simulink model "SigProcess"  (R2022b)
settings: Solver=FixedStepDiscrete  StartTime=0.0  StopTime=10.0  FixedStep=0.001  RelTol=1e-3
undefined symbols (not defined in the file): cClCddAdc_D_u16ADNum, cClCddAdc_D_u8FilterType, cClCddAdc_D_u8RawValueNum, cTmAfCtrl_Te_s32ShttrPosnColdOnHp
libraries: simulink x132
(part 1 of 7)
settings Model: PacingRate=0.500000  Creator=blue.ge  LastModifiedBy=blue.ge
settings OptimizationCC: DefaultParameterBehavior=Inlined  DefaultUnderspecifiedDataType=single  InlineInvariantSignals=on  EnhancedBackFolding=on  StrengthReduction=on  StateBitsets=on  DataBitsets=on  ZeroExternalMemoryAtStartup=off  ZeroInternalMemoryAtStartup=off  EfficientFloat2IntCast=on  LifeSpan=inf  EfficientTunableParamExpr=on
settings DebuggingCC: ConsistencyChecking=error  SignalInfNanChecking=warning  SignalRangeChecking=warning  AlgebraicLoopMsg=error  ArtificialAlgebraicLoopMsg=error  SaveWithDisabledLinksMsg=none  SaveWithParameterizedLinksMsg=none  SignalResolutionControl=TryResolveAll  BlockPriorityViolationMsg=error  SolverPrmCheckMsg=error  SingleTaskRateTransMsg=error  SigSpecEnsureSampleTimeMsg=error  CheckMatrixSingularityMsg=error  ParameterOverflowMsg=warning  ParameterUnderflowMsg=error  ParameterTunabilityLossMsg=error  UnderSpecifiedDataTypeMsg=warning  UnnecessaryDatatypeConvMsg=warning  VectorMatrixConversionMsg=error  SignalLabelMismatchMsg=warning  UnconnectedLineMsg=error  UniqueDataStoreMsg=error  BusObjectLabelMismatch=error  RootOutportRequireBusObject=error  AllowSymbolicDim=off  ModelReferenceIOMsg=error  ModelReferenceIOMismatchMessage=error  UnknownTsInhSupMsg=error  ModelReferenceDataLoggingMessage=error  ModelReferenceNoExplicitFinalValueMsg=error  StateNameClashWarn=warning  StrictBusMsg=ErrorOnBusTreatedAsVector  NonBusSignalsTreatedAsBus=warning  SFTemporalDelaySmallerThanSampleTimeDiag=error  SFMachineParentedDataDiag=warning  VariantConditionMismatch=warning
settings HardwareCC: ProdBitPerPointer=32  ProdBitPerSizeT=32  ProdBitPerPtrDiffT=32  ProdLargestAtomicInteger=Long  ProdWordSize=32  ProdLongLongMode=on  ProdHWDeviceType=Infineon->TriCore
settings ModelReferenceCC: EnableRefExpFcnMdlSchedulingChecks=on  EnableParallelModelReferenceBuilds=on  ParallelModelReferenceMATLABWorkerInit=Copy Base Workspace  ModelReferenceNumInstancesAllowed=Single  PropagateSignalLabelsOutOfModel=off
settings SFSimCC: MATLABDynamicMemAlloc=off  CustomCodeUndefinedFunction=UseInterfaceOnly
settings RTWCC: Description=AUTOSAR  SystemTargetFile=autosar.tlc  GenCodeOnly=on  TemplateMakefile=ert_default_tmf
settings CodeAppCC: GenerateComments=off  IgnoreCustomStorageClasses=off  MaxIdLength=100  OperatorAnnotations=on  SimulinkDataObjDesc=on  SFDataObjDesc=on  MangleLength=10  CustomSymbolStrGlobalVar=global_$R$N$M  CustomSymbolStrType=$N$R$M  CustomSymbolStrBlkIO=local_$N$M  CustomSymbolStrTmpVar=temp_$N$M  SimulinkBlockComments=off
settings STFCustomTargetCC: TargetLangStandard=C99 (ISO)  MultiwordLength=256  ParMdlRefBuildCompliant=on  CompOptLevelCompliant=on  IncludeMdlTerminateFcn=off  CombineOutputUpdateFcns=on  SuppressErrorStatus=on  ERTCustomFileBanners=on  SupportNonFinite=off  SupportComplex=off  SupportContinuousTime=off  SupportNonInlinedSFcns=off  RemoveResetFunc=on  MATLABClassNameForMDSCustomization=Simulink.SoftwareTarget.ERTCustomization  AutosarCompliant=on  UseToolchainInfoCompliant=on  LookupTableObjectStructAxisOrder=2,1,3,4,...  LUTObjectStructOrderEvenSpacing=Size,Table,Breakpoints  SystemTargetFile=autosar.tlc
settings ERTTargetCC: TargetLangStandard=C99 (ISO)  ConcurrentExecutionCompliant=off  IncludeMdlTerminateFcn=off  SuppressErrorStatus=on  SupportNonFinite=off  SupportComplex=off  ModelStepFunctionPrototypeControlCompliant=off  CPPClassGenCompliant=off  AutosarCompliant=on  LookupTableObjectStructAxisOrder=2,1,3,4,...  LUTObjectStructOrderEvenSpacing=Size,Table,Breakpoints  GenerateASAP2=on  InlinedParameterPlacement=NonHierarchical  ERTCustomFileTemplate=example_file_process.tlc  ERTFilePackagingFormat=Compact  ConvertIfToSwitch=off

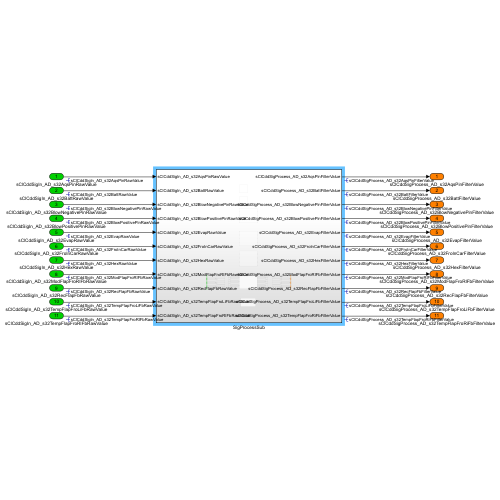
[thumbnail: Simulink's stored preview of the top-level diagram]
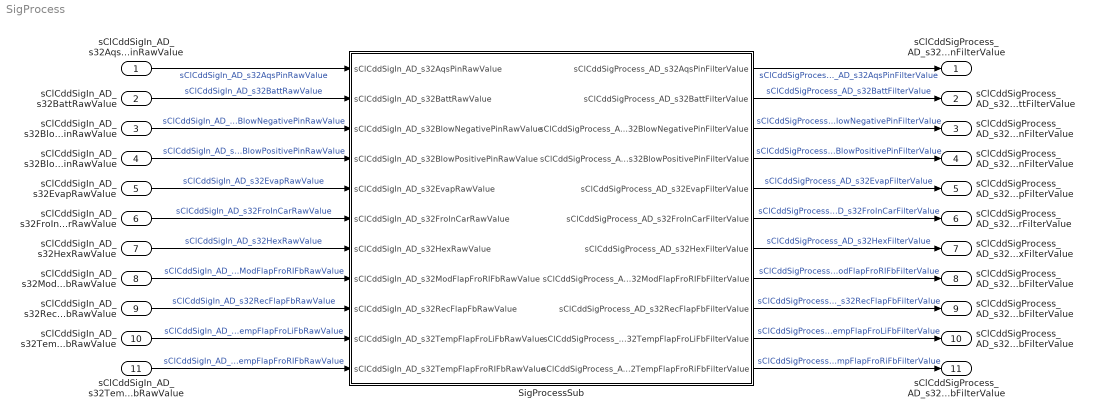
== system SigProcess ==
  sClCddSigIn_AD_s32AqsPinRawValue : Inport  OutDataTypeStr=single
  sClCddSigIn_AD_s32BattRawValue : Inport  Port=2  OutDataTypeStr=single
  sClCddSigIn_AD_s32BlowNegativePinRawValue : Inport  Port=3  OutDataTypeStr=single
  sClCddSigIn_AD_s32BlowPositivePinRawValue : Inport  Port=4  OutDataTypeStr=single
  sClCddSigIn_AD_s32EvapRawValue : Inport  Port=5  OutDataTypeStr=single
  sClCddSigIn_AD_s32FroInCarRawValue : Inport  Port=6  OutDataTypeStr=single
  sClCddSigIn_AD_s32HexRawValue : Inport  Port=7  OutDataTypeStr=single
  sClCddSigIn_AD_s32ModFlapFroRIFbRawValue : Inport  Port=8  OutDataTypeStr=single
  sClCddSigIn_AD_s32RecFlapFbRawValue : Inport  Port=9  OutDataTypeStr=single
  sClCddSigIn_AD_s32TempFlapFroLiFbRawValue : Inport  Port=10  OutDataTypeStr=single
  sClCddSigIn_AD_s32TempFlapFroRIFbRawValue : Inport  Port=11  OutDataTypeStr=single
  SigProcessSub : Subsystem
  sClCddSigProcess_AD_s32AqsPinFilterValue : Outport  OutDataTypeStr=single
  sClCddSigProcess_AD_s32BattFilterValue : Outport  Port=2  OutDataTypeStr=single
  sClCddSigProcess_AD_s32BlowNegativePinFilterValue : Outport  Port=3  OutDataTypeStr=single
  sClCddSigProcess_AD_s32BlowPositivePinFilterValue : Outport  Port=4  OutDataTypeStr=single
  sClCddSigProcess_AD_s32EvapFilterValue : Outport  Port=5  OutDataTypeStr=single
  sClCddSigProcess_AD_s32FroInCarFilterValue : Outport  Port=6  OutDataTypeStr=single
  sClCddSigProcess_AD_s32HexFilterValue : Outport  Port=7  OutDataTypeStr=single
  sClCddSigProcess_AD_s32ModFlapFroRIFbFilterValue : Outport  Port=8  OutDataTypeStr=single
  sClCddSigProcess_AD_s32RecFlapFbFilterValue : Outport  Port=9  OutDataTypeStr=single
  sClCddSigProcess_AD_s32TempFlapFroLiFbFilterValue : Outport  Port=10  OutDataTypeStr=single
  sClCddSigProcess_AD_s32TempFlapFroRiFbFilterValue : Outport  Port=11  OutDataTypeStr=single
  wires:
  sClCddSigIn_AD_s32AqsPinRawValue/1 -> SigProcessSub/1(sClCddSigIn_AD_s32AqsPinRawValue)  "sClCddSigIn_AD_s32AqsPinRawValue"
  sClCddSigIn_AD_s32BattRawValue/1 -> SigProcessSub/2(sClCddSigIn_AD_s32BattRawValue)  "sClCddSigIn_AD_s32BattRawValue"
  sClCddSigIn_AD_s32BlowNegativePinRawValue/1 -> SigProcessSub/3(sClCddSigIn_AD_s32BlowNegativePinRawValue)  "sClCddSigIn_AD_s32BlowNegativePinRawValue"
  sClCddSigIn_AD_s32BlowPositivePinRawValue/1 -> SigProcessSub/4(sClCddSigIn_AD_s32BlowPositivePinRawValue)  "sClCddSigIn_AD_s32BlowPositivePinRawValue"
  sClCddSigIn_AD_s32EvapRawValue/1 -> SigProcessSub/5(sClCddSigIn_AD_s32EvapRawValue)  "sClCddSigIn_AD_s32EvapRawValue"
  sClCddSigIn_AD_s32FroInCarRawValue/1 -> SigProcessSub/6(sClCddSigIn_AD_s32FroInCarRawValue)  "sClCddSigIn_AD_s32FroInCarRawValue"
  sClCddSigIn_AD_s32HexRawValue/1 -> SigProcessSub/7(sClCddSigIn_AD_s32HexRawValue)  "sClCddSigIn_AD_s32HexRawValue"
  sClCddSigIn_AD_s32ModFlapFroRIFbRawValue/1 -> SigProcessSub/8(sClCddSigIn_AD_s32ModFlapFroRIFbRawValue)  "sClCddSigIn_AD_s32ModFlapFroRIFbRawValue"
  sClCddSigIn_AD_s32RecFlapFbRawValue/1 -> SigProcessSub/9(sClCddSigIn_AD_s32RecFlapFbRawValue)  "sClCddSigIn_AD_s32RecFlapFbRawValue"
  sClCddSigIn_AD_s32TempFlapFroLiFbRawValue/1 -> SigProcessSub/10(sClCddSigIn_AD_s32TempFlapFroLiFbRawValue)  "sClCddSigIn_AD_s32TempFlapFroLiFbRawValue"
  sClCddSigIn_AD_s32TempFlapFroRIFbRawValue/1 -> SigProcessSub/11(sClCddSigIn_AD_s32TempFlapFroRIFbRawValue)  "sClCddSigIn_AD_s32TempFlapFroRIFbRawValue"
  SigProcessSub/1(sClCddSigProcess_AD_s32AqsPinFilterValue) -> sClCddSigProcess_AD_s32AqsPinFilterValue/1  "sClCddSigProcess_AD_s32AqsPinFilterValue"
  SigProcessSub/2(sClCddSigProcess_AD_s32BattFilterValue) -> sClCddSigProcess_AD_s32BattFilterValue/1  "sClCddSigProcess_AD_s32BattFilterValue"
  SigProcessSub/3(sClCddSigProcess_AD_s32BlowNegativePinFilterValue) -> sClCddSigProcess_AD_s32BlowNegativePinFilterValue/1  "sClCddSigProcess_AD_s32BlowNegativePinFilterValue"
  SigProcessSub/4(sClCddSigProcess_AD_s32BlowPositivePinFilterValue) -> sClCddSigProcess_AD_s32BlowPositivePinFilterValue/1  "sClCddSigProcess_AD_s32BlowPositivePinFilterValue"
  SigProcessSub/5(sClCddSigProcess_AD_s32EvapFilterValue) -> sClCddSigProcess_AD_s32EvapFilterValue/1  "sClCddSigProcess_AD_s32EvapFilterValue"
  SigProcessSub/6(sClCddSigProcess_AD_s32FroInCarFilterValue) -> sClCddSigProcess_AD_s32FroInCarFilterValue/1  "sClCddSigProcess_AD_s32FroInCarFilterValue"
  SigProcessSub/7(sClCddSigProcess_AD_s32HexFilterValue) -> sClCddSigProcess_AD_s32HexFilterValue/1  "sClCddSigProcess_AD_s32HexFilterValue"
  SigProcessSub/8(sClCddSigProcess_AD_s32ModFlapFroRIFbFilterValue) -> sClCddSigProcess_AD_s32ModFlapFroRIFbFilterValue/1  "sClCddSigProcess_AD_s32ModFlapFroRIFbFilterValue"
  SigProcessSub/9(sClCddSigProcess_AD_s32RecFlapFbFilterValue) -> sClCddSigProcess_AD_s32RecFlapFbFilterValue/1  "sClCddSigProcess_AD_s32RecFlapFbFilterValue"
  SigProcessSub/10(sClCddSigProcess_AD_s32TempFlapFroLiFbFilterValue) -> sClCddSigProcess_AD_s32TempFlapFroLiFbFilterValue/1  "sClCddSigProcess_AD_s32TempFlapFroLiFbFilterValue"
  SigProcessSub/11(sClCddSigProcess_AD_s32TempFlapFroRiFbFilterValue) -> sClCddSigProcess_AD_s32TempFlapFroRiFbFilterValue/1  "sClCddSigProcess_AD_s32TempFlapFroRiFbFilterValue"

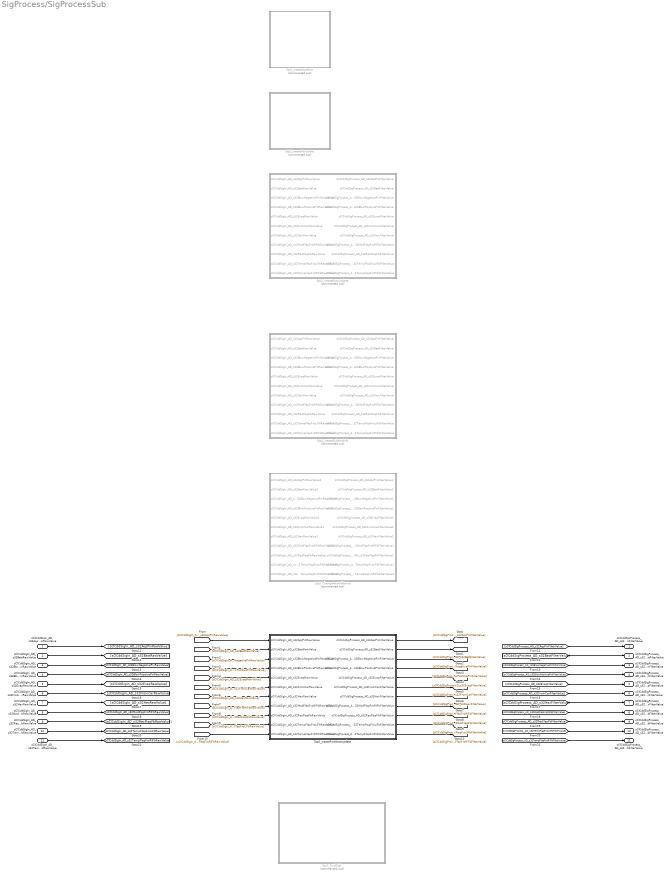
== system SigProcess/SigProcessSub ==
  sClCddSigIn_AD_s32AqsPinRawValue : Inport  OutDataTypeStr=single
  sClCddSigIn_AD_s32BattRawValue : Inport  Port=2  OutDataTypeStr=single
  sClCddSigIn_AD_s32BlowNegativePinRawValue : Inport  Port=3  OutDataTypeStr=single
  sClCddSigIn_AD_s32BlowPositivePinRawValue : Inport  Port=4  OutDataTypeStr=single
  sClCddSigIn_AD_s32EvapRawValue : Inport  Port=5  OutDataTypeStr=single
  sClCddSigIn_AD_s32FroInCarRawValue : Inport  Port=6  OutDataTypeStr=single
  sClCddSigIn_AD_s32HexRawValue : Inport  Port=7  OutDataTypeStr=single
  sClCddSigIn_AD_s32ModFlapFroRIFbRawValue : Inport  Port=8  OutDataTypeStr=single
  sClCddSigIn_AD_s32RecFlapFbRawValue : Inport  Port=9  OutDataTypeStr=single
  sClCddSigIn_AD_s32TempFlapFroLiFbRawValue : Inport  Port=10  OutDataTypeStr=single
  sClCddSigIn_AD_s32TempFlapFroRIFbRawValue : Inport  Port=11  OutDataTypeStr=single
  Stp1_createSubMod : Subsystem  Commented=on
  Stp2_createPortsGoto : Subsystem  Commented=on
  Stp3_createGotoUpdate : Subsystem  Commented=on
  Stp4_createSubModInfo : Subsystem  Commented=on
  Stp5_ChangeAttrAndName : Subsystem  Commented=on
  Stp6_createPortGotoUpdate : Subsystem
  Stp7_FindSldd : Subsystem  Commented=on
  sClCddSigProcess_AD_s32AqsPinFilterValue : Outport  OutDataTypeStr=single
  sClCddSigProcess_AD_s32BattFilterValue : Outport  Port=2  OutDataTypeStr=single
  sClCddSigProcess_AD_s32BlowNegativePinFilterValue : Outport  Port=3  OutDataTypeStr=single
  sClCddSigProcess_AD_s32BlowPositivePinFilterValue : Outport  Port=4  OutDataTypeStr=single
  sClCddSigProcess_AD_s32EvapFilterValue : Outport  Port=5  OutDataTypeStr=single
  sClCddSigProcess_AD_s32FroInCarFilterValue : Outport  Port=6  OutDataTypeStr=single
  sClCddSigProcess_AD_s32HexFilterValue : Outport  Port=7  OutDataTypeStr=single
  sClCddSigProcess_AD_s32ModFlapFroRIFbFilterValue : Outport  Port=8  OutDataTypeStr=single
  sClCddSigProcess_AD_s32RecFlapFbFilterValue : Outport  Port=9  OutDataTypeStr=single
  sClCddSigProcess_AD_s32TempFlapFroLiFbFilterValue : Outport  Port=10  OutDataTypeStr=single
  sClCddSigProcess_AD_s32TempFlapFroRiFbFilterValue : Outport  Port=11  OutDataTypeStr=single
  wires:
  [sClCddSigIn_AD_s32AqsPinRawValue] -> Stp6_createPortGotoUpdate/1(sClCddSigIn_AD_s32AqsPinRawValue)
  [sClCddSigIn_AD_s32BattRawValue] -> Stp6_createPortGotoUpdate/2(sClCddSigIn_AD_s32BattRawValue)
  [sClCddSigIn_AD_s32BlowNegativePinRawValue] -> Stp6_createPortGotoUpdate/3(sClCddSigIn_AD_s32BlowNegativePinRawValue)
  [sClCddSigIn_AD_s32BlowPositivePinRawValue] -> Stp6_createPortGotoUpdate/4(sClCddSigIn_AD_s32BlowPositivePinRawValue)
  [sClCddSigIn_AD_s32EvapRawValue] -> Stp6_createPortGotoUpdate/5(sClCddSigIn_AD_s32EvapRawValue)
  [sClCddSigIn_AD_s32FroInCarRawValue] -> Stp6_createPortGotoUpdate/6(sClCddSigIn_AD_s32FroInCarRawValue)
  [sClCddSigIn_AD_s32HexRawValue] -> Stp6_createPortGotoUpdate/7(sClCddSigIn_AD_s32HexRawValue)
  [sClCddSigIn_AD_s32ModFlapFroRIFbRawValue] -> Stp6_createPortGotoUpdate/8(sClCddSigIn_AD_s32ModFlapFroRIFbRawValue)
  [sClCddSigIn_AD_s32RecFlapFbRawValue] -> Stp6_createPortGotoUpdate/9(sClCddSigIn_AD_s32RecFlapFbRawValue)
  [sClCddSigIn_AD_s32TempFlapFroLiFbRawValue] -> Stp6_createPortGotoUpdate/10(sClCddSigIn_AD_s32TempFlapFroLiFbRawValue)
  [sClCddSigIn_AD_s32TempFlapFroRIFbRawValue] -> Stp6_createPortGotoUpdate/11(sClCddSigIn_AD_s32TempFlapFroRIFbRawValue)
  Stp6_createPortGotoUpdate/1(sClCddSigProcess_AD_s32AqsPinFilterValue) -> [sClCddSigProcess_AD_s32AqsPinFilterValue]
  Stp6_createPortGotoUpdate/2(sClCddSigProcess_AD_s32BattFilterValue) -> [sClCddSigProcess_AD_s32BattFilterValue]
  Stp6_createPortGotoUpdate/3(sClCddSigProcess_AD_s32BlowNegativePinFilterValue) -> [sClCddSigProcess_AD_s32BlowNegativePinFilterValue]
  Stp6_createPortGotoUpdate/4(sClCddSigProcess_AD_s32BlowPositivePinFilterValue) -> [sClCddSigProcess_AD_s32BlowPositivePinFilterValue]
  Stp6_createPortGotoUpdate/5(sClCddSigProcess_AD_s32EvapFilterValue) -> [sClCddSigProcess_AD_s32EvapFilterValue]
  Stp6_createPortGotoUpdate/6(sClCddSigProcess_AD_s32FroInCarFilterValue) -> [sClCddSigProcess_AD_s32FroInCarFilterValue]
  Stp6_createPortGotoUpdate/7(sClCddSigProcess_AD_s32HexFilterValue) -> [sClCddSigProcess_AD_s32HexFilterValue]
  Stp6_createPortGotoUpdate/8(sClCddSigProcess_AD_s32ModFlapFroRIFbFilterValue) -> [sClCddSigProcess_AD_s32ModFlapFroRIFbFilterValue]
  Stp6_createPortGotoUpdate/9(sClCddSigProcess_AD_s32RecFlapFbFilterValue) -> [sClCddSigProcess_AD_s32RecFlapFbFilterValue]
  Stp6_createPortGotoUpdate/10(sClCddSigProcess_AD_s32TempFlapFroLiFbFilterValue) -> [sClCddSigProcess_AD_s32TempFlapFroLiFbFilterValue]
  Stp6_createPortGotoUpdate/11(sClCddSigProcess_AD_s32TempFlapFroRiFbFilterValue) -> [sClCddSigProcess_AD_s32TempFlapFroRiFbFilterValue]
  sClCddSigIn_AD_s32AqsPinRawValue/1 -> [sClCddSigIn_AD_s32AqsPinRawValue]
  sClCddSigIn_AD_s32BattRawValue/1 -> [sClCddSigIn_AD_s32BattRawValue]
  sClCddSigIn_AD_s32BlowNegativePinRawValue/1 -> [sClCddSigIn_AD_s32BlowNegativePinRawValue]
  sClCddSigIn_AD_s32BlowPositivePinRawValue/1 -> [sClCddSigIn_AD_s32BlowPositivePinRawValue]
  sClCddSigIn_AD_s32EvapRawValue/1 -> [sClCddSigIn_AD_s32EvapRawValue]
  sClCddSigIn_AD_s32FroInCarRawValue/1 -> [sClCddSigIn_AD_s32FroInCarRawValue]
  sClCddSigIn_AD_s32HexRawValue/1 -> [sClCddSigIn_AD_s32HexRawValue]
  sClCddSigIn_AD_s32ModFlapFroRIFbRawValue/1 -> [sClCddSigIn_AD_s32ModFlapFroRIFbRawValue]
  sClCddSigIn_AD_s32RecFlapFbRawValue/1 -> [sClCddSigIn_AD_s32RecFlapFbRawValue]
  sClCddSigIn_AD_s32TempFlapFroLiFbRawValue/1 -> [sClCddSigIn_AD_s32TempFlapFroLiFbRawValue]
  sClCddSigIn_AD_s32TempFlapFroRIFbRawValue/1 -> [sClCddSigIn_AD_s32TempFlapFroRIFbRawValue]
  [sClCddSigProcess_AD_s32AqsPinFilterValue] -> sClCddSigProcess_AD_s32AqsPinFilterValue/1
  [sClCddSigProcess_AD_s32BattFilterValue] -> sClCddSigProcess_AD_s32BattFilterValue/1
  [sClCddSigProcess_AD_s32BlowNegativePinFilterValue] -> sClCddSigProcess_AD_s32BlowNegativePinFilterValue/1
  [sClCddSigProcess_AD_s32BlowPositivePinFilterValue] -> sClCddSigProcess_AD_s32BlowPositivePinFilterValue/1
  [sClCddSigProcess_AD_s32EvapFilterValue] -> sClCddSigProcess_AD_s32EvapFilterValue/1
  [sClCddSigProcess_AD_s32FroInCarFilterValue] -> sClCddSigProcess_AD_s32FroInCarFilterValue/1
  [sClCddSigProcess_AD_s32HexFilterValue] -> sClCddSigProcess_AD_s32HexFilterValue/1
  [sClCddSigProcess_AD_s32ModFlapFroRIFbFilterValue] -> sClCddSigProcess_AD_s32ModFlapFroRIFbFilterValue/1
  [sClCddSigProcess_AD_s32RecFlapFbFilterValue] -> sClCddSigProcess_AD_s32RecFlapFbFilterValue/1
  [sClCddSigProcess_AD_s32TempFlapFroLiFbFilterValue] -> sClCddSigProcess_AD_s32TempFlapFroLiFbFilterValue/1
  [sClCddSigProcess_AD_s32TempFlapFroRiFbFilterValue] -> sClCddSigProcess_AD_s32TempFlapFroRiFbFilterValue/1

== system SigProcess/SigProcessSub/Stp1_createSubMod ==
  CLHB02001_AdFilter : Subsystem
  CLHB02001_AdVoltChange : Subsystem

== system SigProcess/SigProcessSub/Stp2_createPortsGoto ==
  CLHB02001_AdFilter : Subsystem
  CLHB02001_AdVoltChange : Subsystem

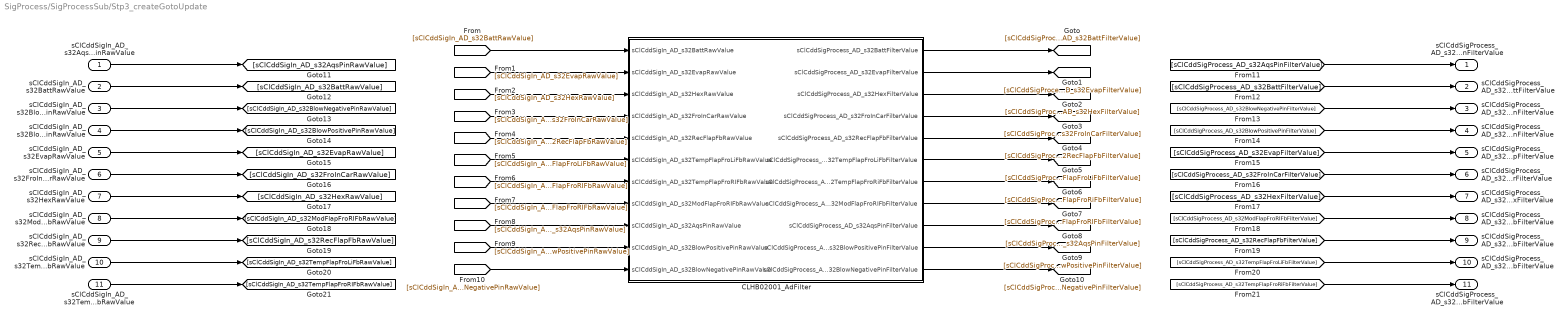
== system SigProcess/SigProcessSub/Stp3_createGotoUpdate ==
  sClCddSigIn_AD_s32AqsPinRawValue : Inport  OutDataTypeStr=single
  sClCddSigIn_AD_s32BattRawValue : Inport  Port=2  OutDataTypeStr=single
  sClCddSigIn_AD_s32BlowNegativePinRawValue : Inport  Port=3  OutDataTypeStr=single
  sClCddSigIn_AD_s32BlowPositivePinRawValue : Inport  Port=4  OutDataTypeStr=single
  sClCddSigIn_AD_s32EvapRawValue : Inport  Port=5  OutDataTypeStr=single
  sClCddSigIn_AD_s32FroInCarRawValue : Inport  Port=6  OutDataTypeStr=single
  sClCddSigIn_AD_s32HexRawValue : Inport  Port=7  OutDataTypeStr=single
  sClCddSigIn_AD_s32ModFlapFroRIFbRawValue : Inport  Port=8  OutDataTypeStr=single
  sClCddSigIn_AD_s32RecFlapFbRawValue : Inport  Port=9  OutDataTypeStr=single
  sClCddSigIn_AD_s32TempFlapFroLiFbRawValue : Inport  Port=10  OutDataTypeStr=single
  sClCddSigIn_AD_s32TempFlapFroRIFbRawValue : Inport  Port=11  OutDataTypeStr=single
  CLHB02001_AdFilter : Subsystem
  sClCddSigProcess_AD_s32AqsPinFilterValue : Outport  OutDataTypeStr=single
  sClCddSigProcess_AD_s32BattFilterValue : Outport  Port=2  OutDataTypeStr=single
  sClCddSigProcess_AD_s32BlowNegativePinFilterValue : Outport  Port=3  OutDataTypeStr=single
  sClCddSigProcess_AD_s32BlowPositivePinFilterValue : Outport  Port=4  OutDataTypeStr=single
  sClCddSigProcess_AD_s32EvapFilterValue : Outport  Port=5  OutDataTypeStr=single
  sClCddSigProcess_AD_s32FroInCarFilterValue : Outport  Port=6  OutDataTypeStr=single
  sClCddSigProcess_AD_s32HexFilterValue : Outport  Port=7  OutDataTypeStr=single
  sClCddSigProcess_AD_s32ModFlapFroRIFbFilterValue : Outport  Port=8  OutDataTypeStr=single
  sClCddSigProcess_AD_s32RecFlapFbFilterValue : Outport  Port=9  OutDataTypeStr=single
  sClCddSigProcess_AD_s32TempFlapFroLiFbFilterValue : Outport  Port=10  OutDataTypeStr=single
  sClCddSigProcess_AD_s32TempFlapFroRiFbFilterValue : Outport  Port=11  OutDataTypeStr=single
  wires:
  [sClCddSigIn_AD_s32BattRawValue] -> CLHB02001_AdFilter/1(sClCddSigIn_AD_s32BattRawValue)
  [sClCddSigIn_AD_s32EvapRawValue] -> CLHB02001_AdFilter/2(sClCddSigIn_AD_s32EvapRawValue)
  [sClCddSigIn_AD_s32HexRawValue] -> CLHB02001_AdFilter/3(sClCddSigIn_AD_s32HexRawValue)
  [sClCddSigIn_AD_s32FroInCarRawValue] -> CLHB02001_AdFilter/4(sClCddSigIn_AD_s32FroInCarRawValue)
  [sClCddSigIn_AD_s32RecFlapFbRawValue] -> CLHB02001_AdFilter/5(sClCddSigIn_AD_s32RecFlapFbRawValue)
  [sClCddSigIn_AD_s32TempFlapFroLiFbRawValue] -> CLHB02001_AdFilter/6(sClCddSigIn_AD_s32TempFlapFroLiFbRawValue)
  [sClCddSigIn_AD_s32TempFlapFroRIFbRawValue] -> CLHB02001_AdFilter/7(sClCddSigIn_AD_s32TempFlapFroRIFbRawValue)
  [sClCddSigIn_AD_s32ModFlapFroRIFbRawValue] -> CLHB02001_AdFilter/8(sClCddSigIn_AD_s32ModFlapFroRIFbRawValue)
  [sClCddSigIn_AD_s32AqsPinRawValue] -> CLHB02001_AdFilter/9(sClCddSigIn_AD_s32AqsPinRawValue)
  [sClCddSigIn_AD_s32BlowPositivePinRawValue] -> CLHB02001_AdFilter/10(sClCddSigIn_AD_s32BlowPositivePinRawValue)
  [sClCddSigIn_AD_s32BlowNegativePinRawValue] -> CLHB02001_AdFilter/11(sClCddSigIn_AD_s32BlowNegativePinRawValue)
  CLHB02001_AdFilter/1(sClCddSigProcess_AD_s32BattFilterValue) -> [sClCddSigProcess_AD_s32BattFilterValue]
  CLHB02001_AdFilter/2(sClCddSigProcess_AD_s32EvapFilterValue) -> [sClCddSigProcess_AD_s32EvapFilterValue]
  CLHB02001_AdFilter/3(sClCddSigProcess_AD_s32HexFilterValue) -> [sClCddSigProcess_AD_s32HexFilterValue]
  CLHB02001_AdFilter/4(sClCddSigProcess_AD_s32FroInCarFilterValue) -> [sClCddSigProcess_AD_s32FroInCarFilterValue]
  CLHB02001_AdFilter/5(sClCddSigProcess_AD_s32RecFlapFbFilterValue) -> [sClCddSigProcess_AD_s32RecFlapFbFilterValue]
  CLHB02001_AdFilter/6(sClCddSigProcess_AD_s32TempFlapFroLiFbFilterValue) -> [sClCddSigProcess_AD_s32TempFlapFroLiFbFilterValue]
  CLHB02001_AdFilter/7(sClCddSigProcess_AD_s32TempFlapFroRiFbFilterValue) -> [sClCddSigProcess_AD_s32TempFlapFroRiFbFilterValue]
  CLHB02001_AdFilter/8(sClCddSigProcess_AD_s32ModFlapFroRIFbFilterValue) -> [sClCddSigProcess_AD_s32ModFlapFroRIFbFilterValue]
  CLHB02001_AdFilter/9(sClCddSigProcess_AD_s32AqsPinFilterValue) -> [sClCddSigProcess_AD_s32AqsPinFilterValue]
  CLHB02001_AdFilter/10(sClCddSigProcess_AD_s32BlowPositivePinFilterValue) -> [sClCddSigProcess_AD_s32BlowPositivePinFilterValue]
  CLHB02001_AdFilter/11(sClCddSigProcess_AD_s32BlowNegativePinFilterValue) -> [sClCddSigProcess_AD_s32BlowNegativePinFilterValue]
  sClCddSigIn_AD_s32AqsPinRawValue/1 -> [sClCddSigIn_AD_s32AqsPinRawValue]
  sClCddSigIn_AD_s32BattRawValue/1 -> [sClCddSigIn_AD_s32BattRawValue]
  sClCddSigIn_AD_s32BlowNegativePinRawValue/1 -> [sClCddSigIn_AD_s32BlowNegativePinRawValue]
  sClCddSigIn_AD_s32BlowPositivePinRawValue/1 -> [sClCddSigIn_AD_s32BlowPositivePinRawValue]
  sClCddSigIn_AD_s32EvapRawValue/1 -> [sClCddSigIn_AD_s32EvapRawValue]
  sClCddSigIn_AD_s32FroInCarRawValue/1 -> [sClCddSigIn_AD_s32FroInCarRawValue]
  sClCddSigIn_AD_s32HexRawValue/1 -> [sClCddSigIn_AD_s32HexRawValue]
  sClCddSigIn_AD_s32ModFlapFroRIFbRawValue/1 -> [sClCddSigIn_AD_s32ModFlapFroRIFbRawValue]
  sClCddSigIn_AD_s32RecFlapFbRawValue/1 -> [sClCddSigIn_AD_s32RecFlapFbRawValue]
  sClCddSigIn_AD_s32TempFlapFroLiFbRawValue/1 -> [sClCddSigIn_AD_s32TempFlapFroLiFbRawValue]
  sClCddSigIn_AD_s32TempFlapFroRIFbRawValue/1 -> [sClCddSigIn_AD_s32TempFlapFroRIFbRawValue]
  [sClCddSigProcess_AD_s32AqsPinFilterValue] -> sClCddSigProcess_AD_s32AqsPinFilterValue/1
  [sClCddSigProcess_AD_s32BattFilterValue] -> sClCddSigProcess_AD_s32BattFilterValue/1
  [sClCddSigProcess_AD_s32BlowNegativePinFilterValue] -> sClCddSigProcess_AD_s32BlowNegativePinFilterValue/1
  [sClCddSigProcess_AD_s32BlowPositivePinFilterValue] -> sClCddSigProcess_AD_s32BlowPositivePinFilterValue/1
  [sClCddSigProcess_AD_s32EvapFilterValue] -> sClCddSigProcess_AD_s32EvapFilterValue/1
  [sClCddSigProcess_AD_s32FroInCarFilterValue] -> sClCddSigProcess_AD_s32FroInCarFilterValue/1
  [sClCddSigProcess_AD_s32HexFilterValue] -> sClCddSigProcess_AD_s32HexFilterValue/1
  [sClCddSigProcess_AD_s32ModFlapFroRIFbFilterValue] -> sClCddSigProcess_AD_s32ModFlapFroRIFbFilterValue/1
  [sClCddSigProcess_AD_s32RecFlapFbFilterValue] -> sClCddSigProcess_AD_s32RecFlapFbFilterValue/1
  [sClCddSigProcess_AD_s32TempFlapFroLiFbFilterValue] -> sClCddSigProcess_AD_s32TempFlapFroLiFbFilterValue/1
  [sClCddSigProcess_AD_s32TempFlapFroRiFbFilterValue] -> sClCddSigProcess_AD_s32TempFlapFroRiFbFilterValue/1

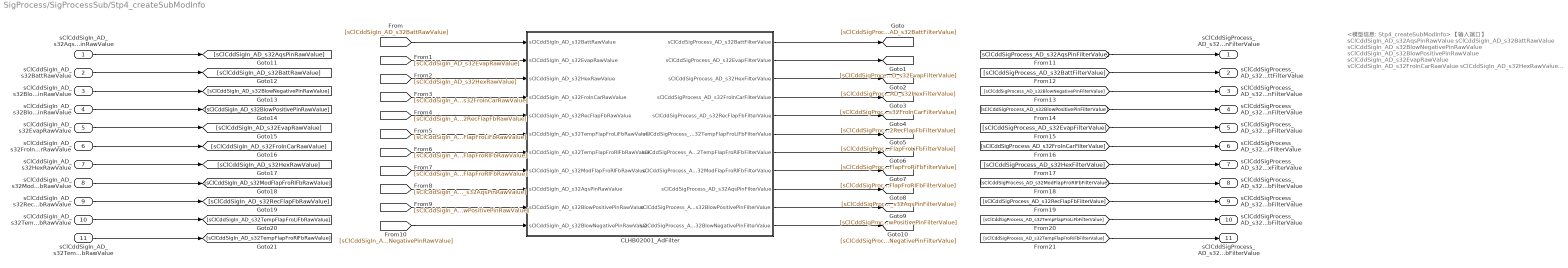
== system SigProcess/SigProcessSub/Stp4_createSubModInfo ==
  note: <模型信息: Stp4_createSubModInfo>
      |
      |
      | 【输入端口】
      | sClCddSigIn_AD_s32AqsPinRawValue
      | sClCddSigIn_AD_s32BattRawValue
      | sClCddSigIn_AD_s32BlowNegativePinRawValue
      | sClCddSigIn_AD_s32BlowPositivePinRawValue
      | sClCddSigIn_AD_s32EvapRawValue
      | sClCddSigIn_AD_s32FroInCarRawValue
      | sClCddSigIn_AD_s32HexRawValue
      | sClCddSigIn_AD_s32ModFlapFroRIFbRawValue
      | sClCddSigIn_AD_s32RecFlapFbRawValue
      | sClCddSigIn_AD_s32TempFlapFroLiFbRawValue
      | sClCddSigIn_AD_s32TempFlapFroRIFbRawValue
      |
      | 【输出端口】
      | sClCddSigProcess_AD_s32AqsPinFilterValue
      | sClCddSigProcess_AD_s32BattFilterValue
      | sClCddSigProcess_AD_s32BlowNegativePinFilterValue
      | sClCddSigProcess_AD_s32BlowPositivePinFilterValue
      | sClCddSigProcess_AD_s32EvapFilterValue
      | sClCddSigProcess_AD_s32FroInCarFilterValue
      | sClCddSigProcess_AD_s32HexFilterValue
      | sClCddSigProcess_AD_s32ModFlapFroRIFbFilterValue
      | sClCddSigProcess_AD_s32RecFlapFbFilterValue
      | sClCddSigProcess_AD_s32TempFlapFroLiFbFilterValue
      | sClCddSigProcess_AD_s32TempFlapFroRiFbFilterValue
      |
      | 【标定量】
      | 无标定量
      |
      | 创建时间: 2025-06-10 10:15:24
  sClCddSigIn_AD_s32AqsPinRawValue : Inport  OutDataTypeStr=single
  sClCddSigIn_AD_s32BattRawValue : Inport  Port=2  OutDataTypeStr=single
  sClCddSigIn_AD_s32BlowNegativePinRawValue : Inport  Port=3  OutDataTypeStr=single
  sClCddSigIn_AD_s32BlowPositivePinRawValue : Inport  Port=4  OutDataTypeStr=single
  sClCddSigIn_AD_s32EvapRawValue : Inport  Port=5  OutDataTypeStr=single
  sClCddSigIn_AD_s32FroInCarRawValue : Inport  Port=6  OutDataTypeStr=single
  sClCddSigIn_AD_s32HexRawValue : Inport  Port=7  OutDataTypeStr=single
  sClCddSigIn_AD_s32ModFlapFroRIFbRawValue : Inport  Port=8  OutDataTypeStr=single
  sClCddSigIn_AD_s32RecFlapFbRawValue : Inport  Port=9  OutDataTypeStr=single
  sClCddSigIn_AD_s32TempFlapFroLiFbRawValue : Inport  Port=10  OutDataTypeStr=single
  sClCddSigIn_AD_s32TempFlapFroRIFbRawValue : Inport  Port=11  OutDataTypeStr=single
  CLHB02001_AdFilter : Subsystem
  sClCddSigProcess_AD_s32AqsPinFilterValue : Outport  OutDataTypeStr=single
  sClCddSigProcess_AD_s32BattFilterValue : Outport  Port=2  OutDataTypeStr=single
  sClCddSigProcess_AD_s32BlowNegativePinFilterValue : Outport  Port=3  OutDataTypeStr=single
  sClCddSigProcess_AD_s32BlowPositivePinFilterValue : Outport  Port=4  OutDataTypeStr=single
  sClCddSigProcess_AD_s32EvapFilterValue : Outport  Port=5  OutDataTypeStr=single
  sClCddSigProcess_AD_s32FroInCarFilterValue : Outport  Port=6  OutDataTypeStr=single
  sClCddSigProcess_AD_s32HexFilterValue : Outport  Port=7  OutDataTypeStr=single
  sClCddSigProcess_AD_s32ModFlapFroRIFbFilterValue : Outport  Port=8  OutDataTypeStr=single
  sClCddSigProcess_AD_s32RecFlapFbFilterValue : Outport  Port=9  OutDataTypeStr=single
  sClCddSigProcess_AD_s32TempFlapFroLiFbFilterValue : Outport  Port=10  OutDataTypeStr=single
  sClCddSigProcess_AD_s32TempFlapFroRiFbFilterValue : Outport  Port=11  OutDataTypeStr=single
  wires:
  [sClCddSigIn_AD_s32BattRawValue] -> CLHB02001_AdFilter/1(sClCddSigIn_AD_s32BattRawValue)
  [sClCddSigIn_AD_s32EvapRawValue] -> CLHB02001_AdFilter/2(sClCddSigIn_AD_s32EvapRawValue)
  [sClCddSigIn_AD_s32HexRawValue] -> CLHB02001_AdFilter/3(sClCddSigIn_AD_s32HexRawValue)
  [sClCddSigIn_AD_s32FroInCarRawValue] -> CLHB02001_AdFilter/4(sClCddSigIn_AD_s32FroInCarRawValue)
  [sClCddSigIn_AD_s32RecFlapFbRawValue] -> CLHB02001_AdFilter/5(sClCddSigIn_AD_s32RecFlapFbRawValue)
  [sClCddSigIn_AD_s32TempFlapFroLiFbRawValue] -> CLHB02001_AdFilter/6(sClCddSigIn_AD_s32TempFlapFroLiFbRawValue)
  [sClCddSigIn_AD_s32TempFlapFroRIFbRawValue] -> CLHB02001_AdFilter/7(sClCddSigIn_AD_s32TempFlapFroRIFbRawValue)
  [sClCddSigIn_AD_s32ModFlapFroRIFbRawValue] -> CLHB02001_AdFilter/8(sClCddSigIn_AD_s32ModFlapFroRIFbRawValue)
  [sClCddSigIn_AD_s32AqsPinRawValue] -> CLHB02001_AdFilter/9(sClCddSigIn_AD_s32AqsPinRawValue)
  [sClCddSigIn_AD_s32BlowPositivePinRawValue] -> CLHB02001_AdFilter/10(sClCddSigIn_AD_s32BlowPositivePinRawValue)
  [sClCddSigIn_AD_s32BlowNegativePinRawValue] -> CLHB02001_AdFilter/11(sClCddSigIn_AD_s32BlowNegativePinRawValue)
  CLHB02001_AdFilter/1(sClCddSigProcess_AD_s32BattFilterValue) -> [sClCddSigProcess_AD_s32BattFilterValue]
  CLHB02001_AdFilter/2(sClCddSigProcess_AD_s32EvapFilterValue) -> [sClCddSigProcess_AD_s32EvapFilterValue]
  CLHB02001_AdFilter/3(sClCddSigProcess_AD_s32HexFilterValue) -> [sClCddSigProcess_AD_s32HexFilterValue]
  CLHB02001_AdFilter/4(sClCddSigProcess_AD_s32FroInCarFilterValue) -> [sClCddSigProcess_AD_s32FroInCarFilterValue]
  CLHB02001_AdFilter/5(sClCddSigProcess_AD_s32RecFlapFbFilterValue) -> [sClCddSigProcess_AD_s32RecFlapFbFilterValue]
  CLHB02001_AdFilter/6(sClCddSigProcess_AD_s32TempFlapFroLiFbFilterValue) -> [sClCddSigProcess_AD_s32TempFlapFroLiFbFilterValue]
  CLHB02001_AdFilter/7(sClCddSigProcess_AD_s32TempFlapFroRiFbFilterValue) -> [sClCddSigProcess_AD_s32TempFlapFroRiFbFilterValue]
  CLHB02001_AdFilter/8(sClCddSigProcess_AD_s32ModFlapFroRIFbFilterValue) -> [sClCddSigProcess_AD_s32ModFlapFroRIFbFilterValue]
  CLHB02001_AdFilter/9(sClCddSigProcess_AD_s32AqsPinFilterValue) -> [sClCddSigProcess_AD_s32AqsPinFilterValue]
  CLHB02001_AdFilter/10(sClCddSigProcess_AD_s32BlowPositivePinFilterValue) -> [sClCddSigProcess_AD_s32BlowPositivePinFilterValue]
  CLHB02001_AdFilter/11(sClCddSigProcess_AD_s32BlowNegativePinFilterValue) -> [sClCddSigProcess_AD_s32BlowNegativePinFilterValue]
  sClCddSigIn_AD_s32AqsPinRawValue/1 -> [sClCddSigIn_AD_s32AqsPinRawValue]
  sClCddSigIn_AD_s32BattRawValue/1 -> [sClCddSigIn_AD_s32BattRawValue]
  sClCddSigIn_AD_s32BlowNegativePinRawValue/1 -> [sClCddSigIn_AD_s32BlowNegativePinRawValue]
  sClCddSigIn_AD_s32BlowPositivePinRawValue/1 -> [sClCddSigIn_AD_s32BlowPositivePinRawValue]
  sClCddSigIn_AD_s32EvapRawValue/1 -> [sClCddSigIn_AD_s32EvapRawValue]
  sClCddSigIn_AD_s32FroInCarRawValue/1 -> [sClCddSigIn_AD_s32FroInCarRawValue]
  sClCddSigIn_AD_s32HexRawValue/1 -> [sClCddSigIn_AD_s32HexRawValue]
  sClCddSigIn_AD_s32ModFlapFroRIFbRawValue/1 -> [sClCddSigIn_AD_s32ModFlapFroRIFbRawValue]
  sClCddSigIn_AD_s32RecFlapFbRawValue/1 -> [sClCddSigIn_AD_s32RecFlapFbRawValue]
  sClCddSigIn_AD_s32TempFlapFroLiFbRawValue/1 -> [sClCddSigIn_AD_s32TempFlapFroLiFbRawValue]
  sClCddSigIn_AD_s32TempFlapFroRIFbRawValue/1 -> [sClCddSigIn_AD_s32TempFlapFroRIFbRawValue]
  [sClCddSigProcess_AD_s32AqsPinFilterValue] -> sClCddSigProcess_AD_s32AqsPinFilterValue/1
  [sClCddSigProcess_AD_s32BattFilterValue] -> sClCddSigProcess_AD_s32BattFilterValue/1
  [sClCddSigProcess_AD_s32BlowNegativePinFilterValue] -> sClCddSigProcess_AD_s32BlowNegativePinFilterValue/1
  [sClCddSigProcess_AD_s32BlowPositivePinFilterValue] -> sClCddSigProcess_AD_s32BlowPositivePinFilterValue/1
  [sClCddSigProcess_AD_s32EvapFilterValue] -> sClCddSigProcess_AD_s32EvapFilterValue/1
  [sClCddSigProcess_AD_s32FroInCarFilterValue] -> sClCddSigProcess_AD_s32FroInCarFilterValue/1
  [sClCddSigProcess_AD_s32HexFilterValue] -> sClCddSigProcess_AD_s32HexFilterValue/1
  [sClCddSigProcess_AD_s32ModFlapFroRIFbFilterValue] -> sClCddSigProcess_AD_s32ModFlapFroRIFbFilterValue/1
  [sClCddSigProcess_AD_s32RecFlapFbFilterValue] -> sClCddSigProcess_AD_s32RecFlapFbFilterValue/1
  [sClCddSigProcess_AD_s32TempFlapFroLiFbFilterValue] -> sClCddSigProcess_AD_s32TempFlapFroLiFbFilterValue/1
  [sClCddSigProcess_AD_s32TempFlapFroRiFbFilterValue] -> sClCddSigProcess_AD_s32TempFlapFroRiFbFilterValue/1

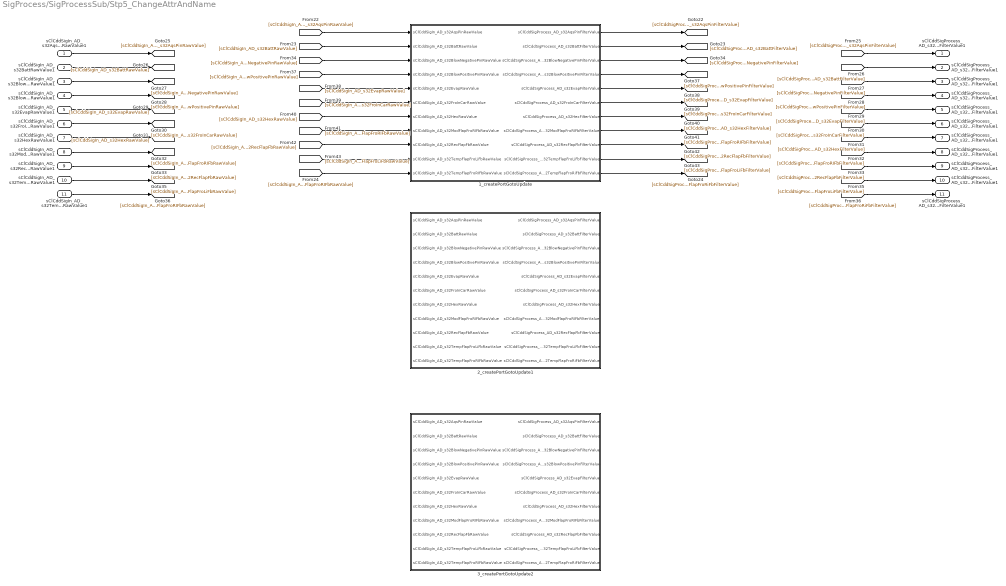
== system SigProcess/SigProcessSub/Stp5_ChangeAttrAndName ==
  sClCddSigIn_AD_s32AqsPinRawValue1 : Inport  OutDataTypeStr=single
  sClCddSigIn_AD_s32BattRawValue1 : Inport  Port=2  OutDataTypeStr=single
  sClCddSigIn_AD_s32BlowNegativePinRawValue1 : Inport  Port=3  OutDataTypeStr=single
  sClCddSigIn_AD_s32BlowPositivePinRawValue1 : Inport  Port=4  OutDataTypeStr=single
  sClCddSigIn_AD_s32EvapRawValue1 : Inport  Port=5  OutDataTypeStr=single
  sClCddSigIn_AD_s32FroInCarRawValue1 : Inport  Port=6  OutDataTypeStr=single
  sClCddSigIn_AD_s32HexRawValue1 : Inport  Port=7  OutDataTypeStr=single
  sClCddSigIn_AD_s32ModFlapFroRIFbRawValue1 : Inport  Port=8  OutDataTypeStr=single
  sClCddSigIn_AD_s32RecFlapFbRawValue1 : Inport  Port=9  OutDataTypeStr=single
  sClCddSigIn_AD_s32TempFlapFroLiFbRawValue1 : Inport  Port=10  OutDataTypeStr=single
  sClCddSigIn_AD_s32TempFlapFroRIFbRawValue1 : Inport  Port=11  OutDataTypeStr=single
  1_createPortGotoUpdate : Subsystem
  2_createPortGotoUpdate1 : Subsystem
  3_createPortGotoUpdate2 : Subsystem
  sClCddSigProcess_AD_s32AqsPinFilterValue1 : Outport  OutDataTypeStr=single
  sClCddSigProcess_AD_s32BattFilterValue1 : Outport  Port=2  OutDataTypeStr=single
  sClCddSigProcess_AD_s32BlowNegativePinFilterValue1 : Outport  Port=3  OutDataTypeStr=single
  sClCddSigProcess_AD_s32BlowPositivePinFilterValue1 : Outport  Port=4  OutDataTypeStr=single
  sClCddSigProcess_AD_s32EvapFilterValue1 : Outport  Port=5  OutDataTypeStr=single
  sClCddSigProcess_AD_s32FroInCarFilterValue1 : Outport  Port=6  OutDataTypeStr=single
  sClCddSigProcess_AD_s32HexFilterValue1 : Outport  Port=7  OutDataTypeStr=single
  sClCddSigProcess_AD_s32ModFlapFroRIFbFilterValue1 : Outport  Port=8  OutDataTypeStr=single
  sClCddSigProcess_AD_s32RecFlapFbFilterValue1 : Outport  Port=9  OutDataTypeStr=single
  sClCddSigProcess_AD_s32TempFlapFroLiFbFilterValue1 : Outport  Port=10  OutDataTypeStr=single
  sClCddSigProcess_AD_s32TempFlapFroRiFbFilterValue1 : Outport  Port=11  OutDataTypeStr=single
  wires:
  [sClCddSigProcess_AD_s32EvapFilterValue] -> sClCddSigProcess_AD_s32EvapFilterValue1/1
  [sClCddSigProcess_AD_s32HexFilterValue] -> sClCddSigProcess_AD_s32HexFilterValue1/1
  sClCddSigIn_AD_s32AqsPinRawValue1/1 -> [sClCddSigIn_AD_s32AqsPinRawValue]
  sClCddSigIn_AD_s32TempFlapFroRIFbRawValue1/1 -> [sClCddSigIn_AD_s32TempFlapFroRIFbRawValue]
  [sClCddSigProcess_AD_s32BlowNegativePinFilterValue] -> sClCddSigProcess_AD_s32BlowNegativePinFilterValue1/1
  [sClCddSigProcess_AD_s32TempFlapFroLiFbFilterValue] -> sClCddSigProcess_AD_s32TempFlapFroLiFbFilterValue1/1
  [sClCddSigProcess_AD_s32RecFlapFbFilterValue] -> sClCddSigProcess_AD_s32RecFlapFbFilterValue1/1
  1_createPortGotoUpdate/11(sClCddSigProcess_AD_s32TempFlapFroRiFbFilterValue) -> [sClCddSigProcess_AD_s32TempFlapFroRiFbFilterValue]
  1_createPortGotoUpdate/8(sClCddSigProcess_AD_s32ModFlapFroRIFbFilterValue) -> [sClCddSigProcess_AD_s32ModFlapFroRIFbFilterValue]
  [sClCddSigProcess_AD_s32FroInCarFilterValue] -> sClCddSigProcess_AD_s32FroInCarFilterValue1/1
  [sClCddSigProcess_AD_s32BattFilterValue] -> sClCddSigProcess_AD_s32BattFilterValue1/1
  sClCddSigIn_AD_s32ModFlapFroRIFbRawValue1/1 -> [sClCddSigIn_AD_s32ModFlapFroRIFbRawValue]
  [sClCddSigIn_AD_s32AqsPinRawValue] -> 1_createPortGotoUpdate/1(sClCddSigIn_AD_s32AqsPinRawValue)
  sClCddSigIn_AD_s32HexRawValue1/1 -> [sClCddSigIn_AD_s32HexRawValue]
  [sClCddSigIn_AD_s32ModFlapFroRIFbRawValue] -> 1_createPortGotoUpdate/8(sClCddSigIn_AD_s32ModFlapFroRIFbRawValue)
  1_createPortGotoUpdate/10(sClCddSigProcess_AD_s32TempFlapFroLiFbFilterValue) -> [sClCddSigProcess_AD_s32TempFlapFroLiFbFilterValue]
  [sClCddSigIn_AD_s32HexRawValue] -> 1_createPortGotoUpdate/7(sClCddSigIn_AD_s32HexRawValue)
  1_createPortGotoUpdate/6(sClCddSigProcess_AD_s32FroInCarFilterValue) -> [sClCddSigProcess_AD_s32FroInCarFilterValue]
  1_createPortGotoUpdate/9(sClCddSigProcess_AD_s32RecFlapFbFilterValue) -> [sClCddSigProcess_AD_s32RecFlapFbFilterValue]
  1_createPortGotoUpdate/5(sClCddSigProcess_AD_s32EvapFilterValue) -> [sClCddSigProcess_AD_s32EvapFilterValue]
  [sClCddSigProcess_AD_s32BlowPositivePinFilterValue] -> sClCddSigProcess_AD_s32BlowPositivePinFilterValue1/1
  1_createPortGotoUpdate/3(sClCddSigProcess_AD_s32BlowNegativePinFilterValue) -> [sClCddSigProcess_AD_s32BlowNegativePinFilterValue]
  [sClCddSigProcess_AD_s32AqsPinFilterValue] -> sClCddSigProcess_AD_s32AqsPinFilterValue1/1
  1_createPortGotoUpdate/4(sClCddSigProcess_AD_s32BlowPositivePinFilterValue) -> [sClCddSigProcess_AD_s32BlowPositivePinFilterValue]
  sClCddSigIn_AD_s32FroInCarRawValue1/1 -> [sClCddSigIn_AD_s32FroInCarRawValue]
  sClCddSigIn_AD_s32BlowNegativePinRawValue1/1 -> [sClCddSigIn_AD_s32BlowNegativePinRawValue]
  sClCddSigIn_AD_s32BattRawValue1/1 -> [sClCddSigIn_AD_s32BattRawValue]
  sClCddSigIn_AD_s32EvapRawValue1/1 -> [sClCddSigIn_AD_s32EvapRawValue]
  [sClCddSigProcess_AD_s32TempFlapFroRiFbFilterValue] -> sClCddSigProcess_AD_s32TempFlapFroRiFbFilterValue1/1
  sClCddSigIn_AD_s32BlowPositivePinRawValue1/1 -> [sClCddSigIn_AD_s32BlowPositivePinRawValue]
  [sClCddSigIn_AD_s32FroInCarRawValue] -> 1_createPortGotoUpdate/6(sClCddSigIn_AD_s32FroInCarRawValue)
  [sClCddSigIn_AD_s32BlowPositivePinRawValue] -> 1_createPortGotoUpdate/4(sClCddSigIn_AD_s32BlowPositivePinRawValue)
  [sClCddSigIn_AD_s32BlowNegativePinRawValue] -> 1_createPortGotoUpdate/3(sClCddSigIn_AD_s32BlowNegativePinRawValue)
  sClCddSigIn_AD_s32TempFlapFroLiFbRawValue1/1 -> [sClCddSigIn_AD_s32TempFlapFroLiFbRawValue]
  [sClCddSigProcess_AD_s32ModFlapFroRIFbFilterValue] -> sClCddSigProcess_AD_s32ModFlapFroRIFbFilterValue1/1
  [sClCddSigIn_AD_s32TempFlapFroRIFbRawValue] -> 1_createPortGotoUpdate/11(sClCddSigIn_AD_s32TempFlapFroRIFbRawValue)
  1_createPortGotoUpdate/7(sClCddSigProcess_AD_s32HexFilterValue) -> [sClCddSigProcess_AD_s32HexFilterValue]
  [sClCddSigIn_AD_s32TempFlapFroLiFbRawValue] -> 1_createPortGotoUpdate/10(sClCddSigIn_AD_s32TempFlapFroLiFbRawValue)
  1_createPortGotoUpdate/1(sClCddSigProcess_AD_s32AqsPinFilterValue) -> [sClCddSigProcess_AD_s32AqsPinFilterValue]
  1_createPortGotoUpdate/2(sClCddSigProcess_AD_s32BattFilterValue) -> [sClCddSigProcess_AD_s32BattFilterValue]
  [sClCddSigIn_AD_s32RecFlapFbRawValue] -> 1_createPortGotoUpdate/9(sClCddSigIn_AD_s32RecFlapFbRawValue)
  sClCddSigIn_AD_s32RecFlapFbRawValue1/1 -> [sClCddSigIn_AD_s32RecFlapFbRawValue]
  [sClCddSigIn_AD_s32BattRawValue] -> 1_createPortGotoUpdate/2(sClCddSigIn_AD_s32BattRawValue)
  [sClCddSigIn_AD_s32EvapRawValue] -> 1_createPortGotoUpdate/5(sClCddSigIn_AD_s32EvapRawValue)

== system SigProcess/SigProcessSub/Stp6_createPortGotoUpdate ==
  note: <模型信息: Stp4_createSubModInfo>
      |
      |
      | 【输入端口】
      | sClCddSigIn_AD_s32AqsPinRawValue
      | sClCddSigIn_AD_s32BattRawValue
      | sClCddSigIn_AD_s32BlowNegativePinRawValue
      | sClCddSigIn_AD_s32BlowPositivePinRawValue
      | sClCddSigIn_AD_s32EvapRawValue
      | sClCddSigIn_AD_s32FroInCarRawValue
      | sClCddSigIn_AD_s32HexRawValue
      | sClCddSigIn_AD_s32ModFlapFroRIFbRawValue
      | sClCddSigIn_AD_s32RecFlapFbRawValue
      | sClCddSigIn_AD_s32TempFlapFroLiFbRawValue
      | sClCddSigIn_AD_s32TempFlapFroRIFbRawValue
      |
      | 【输出端口】
      | sClCddSigProcess_AD_s32AqsPinFilterValue
      | sClCddSigProcess_AD_s32BattFilterValue
      | sClCddSigProcess_AD_s32BlowNegativePinFilterValue
      | sClCddSigProcess_AD_s32BlowPositivePinFilterValue
      | sClCddSigProcess_AD_s32EvapFilterValue
      | sClCddSigProcess_AD_s32FroInCarFilterValue
      | sClCddSigProcess_AD_s32HexFilterValue
      | sClCddSigProcess_AD_s32ModFlapFroRIFbFilterValue
      | sClCddSigProcess_AD_s32RecFlapFbFilterValue
      | sClCddSigProcess_AD_s32TempFlapFroLiFbFilterValue
      | sClCddSigProcess_AD_s32TempFlapFroRiFbFilterValue
      |
      | 【标定量】
      | 无标定量
      |
      | 创建时间: 2025-06-10 10:15:24
  sClCddSigIn_AD_s32AqsPinRawValue : Inport  OutDataTypeStr=single
  sClCddSigIn_AD_s32BattRawValue : Inport  Port=2  OutDataTypeStr=single
  sClCddSigIn_AD_s32BlowNegativePinRawValue : Inport  Port=3  OutDataTypeStr=single
  sClCddSigIn_AD_s32BlowPositivePinRawValue : Inport  Port=4  OutDataTypeStr=single
  sClCddSigIn_AD_s32EvapRawValue : Inport  Port=5  OutDataTypeStr=single
  sClCddSigIn_AD_s32FroInCarRawValue : Inport  Port=6  OutDataTypeStr=single
  sClCddSigIn_AD_s32HexRawValue : Inport  Port=7  OutDataTypeStr=single
  sClCddSigIn_AD_s32ModFlapFroRIFbRawValue : Inport  Port=8  OutDataTypeStr=single
  sClCddSigIn_AD_s32RecFlapFbRawValue : Inport  Port=9  OutDataTypeStr=single
  sClCddSigIn_AD_s32TempFlapFroLiFbRawValue : Inport  Port=10  OutDataTypeStr=single
  sClCddSigIn_AD_s32TempFlapFroRIFbRawValue : Inport  Port=11  OutDataTypeStr=single
  CLHB02001_AdFilter : Subsystem
  sClCddSigProcess_AD_s32AqsPinFilterValue : Outport  OutDataTypeStr=single
  sClCddSigProcess_AD_s32BattFilterValue : Outport  Port=2  OutDataTypeStr=single
  sClCddSigProcess_AD_s32BlowNegativePinFilterValue : Outport  Port=3  OutDataTypeStr=single
  sClCddSigProcess_AD_s32BlowPositivePinFilterValue : Outport  Port=4  OutDataTypeStr=single
  sClCddSigProcess_AD_s32EvapFilterValue : Outport  Port=5  OutDataTypeStr=single
  sClCddSigProcess_AD_s32FroInCarFilterValue : Outport  Port=6  OutDataTypeStr=single
  sClCddSigProcess_AD_s32HexFilterValue : Outport  Port=7  OutDataTypeStr=single
  sClCddSigProcess_AD_s32ModFlapFroRIFbFilterValue : Outport  Port=8  OutDataTypeStr=single
  sClCddSigProcess_AD_s32RecFlapFbFilterValue : Outport  Port=9  OutDataTypeStr=single
  sClCddSigProcess_AD_s32TempFlapFroLiFbFilterValue : Outport  Port=10  OutDataTypeStr=single
  sClCddSigProcess_AD_s32TempFlapFroRiFbFilterValue : Outport  Port=11  OutDataTypeStr=single
  wires:
  [sClCddSigIn_AD_s32BattRawValue] -> CLHB02001_AdFilter/1(sClCddSigIn_AD_s32BattRawValue)
  [sClCddSigIn_AD_s32EvapRawValue] -> CLHB02001_AdFilter/2(sClCddSigIn_AD_s32EvapRawValue)
  [sClCddSigIn_AD_s32HexRawValue] -> CLHB02001_AdFilter/3(sClCddSigIn_AD_s32HexRawValue)
  [sClCddSigIn_AD_s32FroInCarRawValue] -> CLHB02001_AdFilter/4(sClCddSigIn_AD_s32FroInCarRawValue)
  [sClCddSigIn_AD_s32RecFlapFbRawValue] -> CLHB02001_AdFilter/5(sClCddSigIn_AD_s32RecFlapFbRawValue)
  [sClCddSigIn_AD_s32TempFlapFroLiFbRawValue] -> CLHB02001_AdFilter/6(sClCddSigIn_AD_s32TempFlapFroLiFbRawValue)
  [sClCddSigIn_AD_s32TempFlapFroRIFbRawValue] -> CLHB02001_AdFilter/7(sClCddSigIn_AD_s32TempFlapFroRIFbRawValue)
  [sClCddSigIn_AD_s32ModFlapFroRIFbRawValue] -> CLHB02001_AdFilter/8(sClCddSigIn_AD_s32ModFlapFroRIFbRawValue)
  [sClCddSigIn_AD_s32AqsPinRawValue] -> CLHB02001_AdFilter/9(sClCddSigIn_AD_s32AqsPinRawValue)
  [sClCddSigIn_AD_s32BlowPositivePinRawValue] -> CLHB02001_AdFilter/10(sClCddSigIn_AD_s32BlowPositivePinRawValue)
  [sClCddSigIn_AD_s32BlowNegativePinRawValue] -> CLHB02001_AdFilter/11(sClCddSigIn_AD_s32BlowNegativePinRawValue)
  CLHB02001_AdFilter/1(sClCddSigProcess_AD_s32BattFilterValue) -> [sClCddSigProcess_AD_s32BattFilterValue]
  CLHB02001_AdFilter/2(sClCddSigProcess_AD_s32EvapFilterValue) -> [sClCddSigProcess_AD_s32EvapFilterValue]
  CLHB02001_AdFilter/3(sClCddSigProcess_AD_s32HexFilterValue) -> [sClCddSigProcess_AD_s32HexFilterValue]
  CLHB02001_AdFilter/4(sClCddSigProcess_AD_s32FroInCarFilterValue) -> [sClCddSigProcess_AD_s32FroInCarFilterValue]
  CLHB02001_AdFilter/5(sClCddSigProcess_AD_s32RecFlapFbFilterValue) -> [sClCddSigProcess_AD_s32RecFlapFbFilterValue]
  CLHB02001_AdFilter/6(sClCddSigProcess_AD_s32TempFlapFroLiFbFilterValue) -> [sClCddSigProcess_AD_s32TempFlapFroLiFbFilterValue]
  CLHB02001_AdFilter/7(sClCddSigProcess_AD_s32TempFlapFroRiFbFilterValue) -> [sClCddSigProcess_AD_s32TempFlapFroRiFbFilterValue]
  CLHB02001_AdFilter/8(sClCddSigProcess_AD_s32ModFlapFroRIFbFilterValue) -> [sClCddSigProcess_AD_s32ModFlapFroRIFbFilterValue]
  CLHB02001_AdFilter/9(sClCddSigProcess_AD_s32AqsPinFilterValue) -> [sClCddSigProcess_AD_s32AqsPinFilterValue]
  CLHB02001_AdFilter/10(sClCddSigProcess_AD_s32BlowPositivePinFilterValue) -> [sClCddSigProcess_AD_s32BlowPositivePinFilterValue]
  CLHB02001_AdFilter/11(sClCddSigProcess_AD_s32BlowNegativePinFilterValue) -> [sClCddSigProcess_AD_s32BlowNegativePinFilterValue]
  sClCddSigIn_AD_s32AqsPinRawValue/1 -> [sClCddSigIn_AD_s32AqsPinRawValue]
  sClCddSigIn_AD_s32BattRawValue/1 -> [sClCddSigIn_AD_s32BattRawValue]
  sClCddSigIn_AD_s32BlowNegativePinRawValue/1 -> [sClCddSigIn_AD_s32BlowNegativePinRawValue]
  sClCddSigIn_AD_s32BlowPositivePinRawValue/1 -> [sClCddSigIn_AD_s32BlowPositivePinRawValue]
  sClCddSigIn_AD_s32EvapRawValue/1 -> [sClCddSigIn_AD_s32EvapRawValue]
  sClCddSigIn_AD_s32FroInCarRawValue/1 -> [sClCddSigIn_AD_s32FroInCarRawValue]
  sClCddSigIn_AD_s32HexRawValue/1 -> [sClCddSigIn_AD_s32HexRawValue]
  sClCddSigIn_AD_s32ModFlapFroRIFbRawValue/1 -> [sClCddSigIn_AD_s32ModFlapFroRIFbRawValue]
  sClCddSigIn_AD_s32RecFlapFbRawValue/1 -> [sClCddSigIn_AD_s32RecFlapFbRawValue]
  sClCddSigIn_AD_s32TempFlapFroLiFbRawValue/1 -> [sClCddSigIn_AD_s32TempFlapFroLiFbRawValue]
  sClCddSigIn_AD_s32TempFlapFroRIFbRawValue/1 -> [sClCddSigIn_AD_s32TempFlapFroRIFbRawValue]
  [sClCddSigProcess_AD_s32AqsPinFilterValue] -> sClCddSigProcess_AD_s32AqsPinFilterValue/1
  [sClCddSigProcess_AD_s32BattFilterValue] -> sClCddSigProcess_AD_s32BattFilterValue/1
  [sClCddSigProcess_AD_s32BlowNegativePinFilterValue] -> sClCddSigProcess_AD_s32BlowNegativePinFilterValue/1
  [sClCddSigProcess_AD_s32BlowPositivePinFilterValue] -> sClCddSigProcess_AD_s32BlowPositivePinFilterValue/1
  [sClCddSigProcess_AD_s32EvapFilterValue] -> sClCddSigProcess_AD_s32EvapFilterValue/1
  [sClCddSigProcess_AD_s32FroInCarFilterValue] -> sClCddSigProcess_AD_s32FroInCarFilterValue/1
  [sClCddSigProcess_AD_s32HexFilterValue] -> sClCddSigProcess_AD_s32HexFilterValue/1
  [sClCddSigProcess_AD_s32ModFlapFroRIFbFilterValue] -> sClCddSigProcess_AD_s32ModFlapFroRIFbFilterValue/1
  [sClCddSigProcess_AD_s32RecFlapFbFilterValue] -> sClCddSigProcess_AD_s32RecFlapFbFilterValue/1
  [sClCddSigProcess_AD_s32TempFlapFroLiFbFilterValue] -> sClCddSigProcess_AD_s32TempFlapFroLiFbFilterValue/1
  [sClCddSigProcess_AD_s32TempFlapFroRiFbFilterValue] -> sClCddSigProcess_AD_s32TempFlapFroRiFbFilterValue/1

== system SigProcess/SigProcessSub/Stp7_FindSldd ==

== system SigProcess/SigProcessSub/Stp1_createSubMod/CLHB02001_AdFilter ==

== system SigProcess/SigProcessSub/Stp1_createSubMod/CLHB02001_AdVoltChange ==
